simulink model "chap2_8sim"  (Simulink 7.9)
settings: Solver=ode45  SolverMode=SingleTasking  StartTime=0.0  StopTime=20  FixedStep=0.001  RelTol=1e-5  AbsTol=1e-5
settings Model: Creator=liujk  LastModifiedBy=Administrator  ExtModeTrigMode=oneshot  ExtModeArmWhenConnect=off
settings DataIOCC: LimitDataPoints=off
settings OptimizationCC: BlockReduction=off  BooleanDataType=off  ExpressionDepthLimit=128
settings DebuggingCC: SaveWithParameterizedLinksMsg=none  SignalResolutionControl=TryResolveAllWithWarning  SolverPrmCheckMsg=none  MultiTaskDSMMsg=warning  MultiTaskCondExecSysMsg=none  StrictBusMsg=None
settings HardwareCC: TargetUnknown=on
settings RTWCC: IncludeERTFirstTime=on
settings CodeAppCC: CustomSymbolStrType=$N$R$M_T
settings GRTTargetCC: CombineOutputUpdateFcns=off  GRTInterface=on

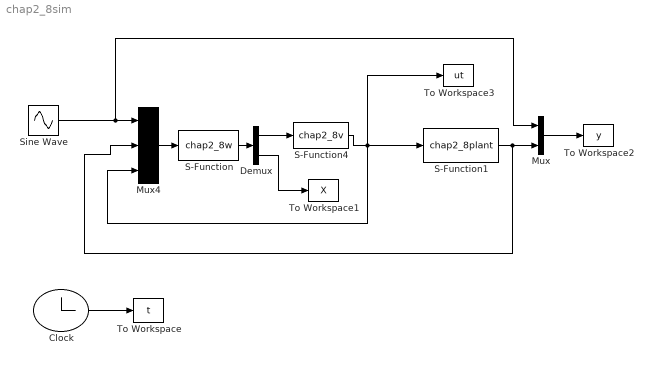
== system chap2_8sim ==
  Clock : Clock
  Demux : Demux  Outputs=2
  Mux : Mux  Inputs=2
  Mux4 : Mux  Inputs=3
  S-Function : S-Function  FunctionName=chap2_8w  EnableBusSupport=off
  S-Function1 : S-Function  FunctionName=chap2_8plant  EnableBusSupport=off
  S-Function4 : S-Function  FunctionName=chap2_8v  EnableBusSupport=off
  Sine Wave : Sin  SampleTime=0
  To Workspace : ToWorkspace  VariableName=t  SampleTime=-1
  To Workspace1 : ToWorkspace  VariableName=X  SampleTime=-1
  To Workspace2 : ToWorkspace  VariableName=y  SampleTime=-1
  To Workspace3 : ToWorkspace  VariableName=ut  SampleTime=-1
  wires:
  Mux4/1 -> S-Function/1
  Mux/1 -> To Workspace2/1
  S-Function1/1 -> Mux/2, Mux4/2
  Sine Wave/1 -> Mux4/1, Mux/1
  Clock/1 -> To Workspace/1
  S-Function4/1 -> Mux4/3, To Workspace3/1, S-Function1/1
  S-Function/1 -> Demux/1
  Demux/1 -> S-Function4/1
  Demux/2 -> To Workspace1/1
